simulink model "control_lab5_sim"  (R2022b)
settings: Solver=VariableStepAuto  StartTime=0.0  StopTime=10.0  RelTol=1e-3
values from neighbouring files (symbols this model uses):
  b = 3.5077e-6    (= 3.5077e-06)    [control_lab5.m]    (also in power_system_1.m = input('Enter any serial number:'))
  J = 3.2284e-6    (= 3.2284e-06)    [control_lab5.m]    (also in newton_rapshon.m = [H,L;M,N;]; newton_rapshon2.m = [H,L;M,N;])
  Ke = 0.0274    [control_lab5.m]
  Kt = 0.000274    [control_lab5.m]
  L = 2^n-1    (= 15)    [PCM__Code.m]    (also in control_lab5.m = 2.75e-06; newton_rapshon.m = zeros(n-1,n-1); newton_rapshon2.m = zeros(n-1,n-1-m))
  R = 19    [control_lab5.m]
settings Model: Creator=Asus  LastModifiedBy=Asus

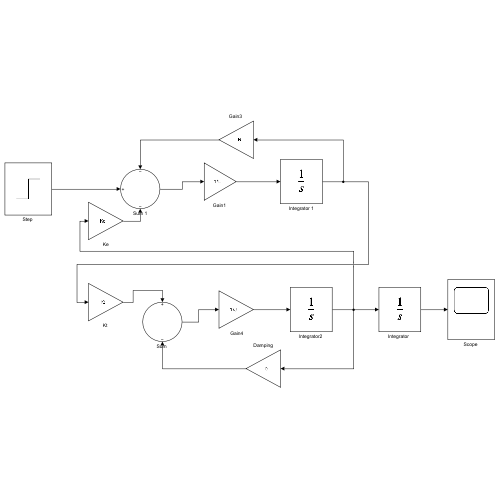
[thumbnail: Simulink's stored preview of the top-level diagram]
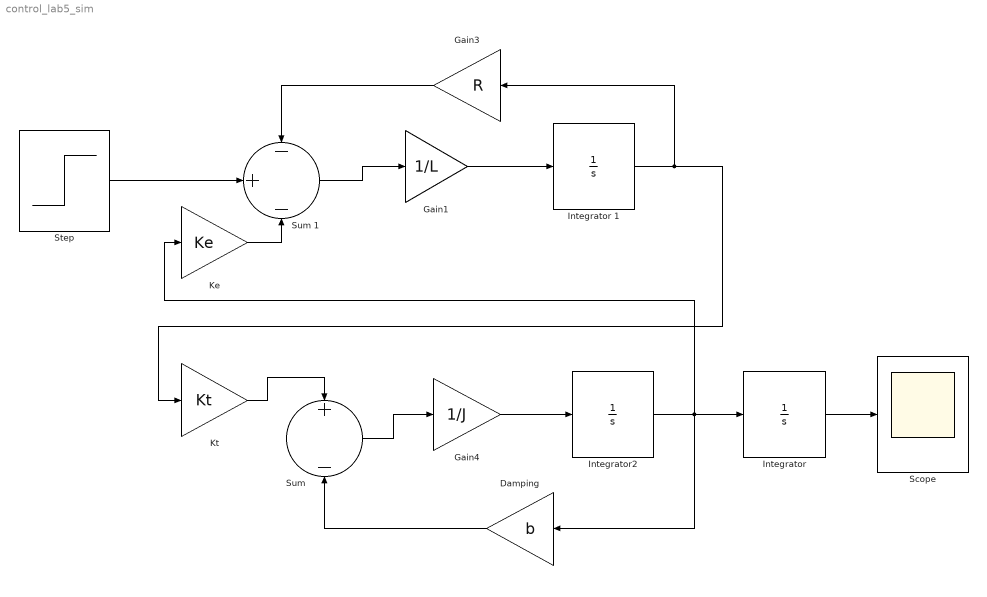
== system control_lab5_sim ==
  " Gain4" : Gain  Gain=1/J
  Damping : Gain  Gain=b
  "Gain1 " : Gain  Gain=1/L
  "Gain3 " : Gain  Gain=R
  "Integrator  " : Integrator
  Integrator 1 : Integrator
  "Integrator2 " : Integrator
  Ke : Gain  Gain=Ke
  "Kt " : Gain  Gain=Kt
  "Scope " : Scope
  "Step " : Step  SampleTime=0
  "Sum " : Sum  Inputs=+-
  Sum 1 : Sum  Inputs=-+-
  wires:
  "Step "/1 -> Sum 1/2
  "Gain3 "/1 -> Sum 1/1
  Ke/1 -> Sum 1/3
  Sum 1/1 -> "Gain1 "/1
  "Gain1 "/1 -> Integrator 1/1
  Integrator 1/1 -> "Kt "/1, "Gain3 "/1
  "Kt "/1 -> "Sum "/1
  Damping/1 -> "Sum "/2
  "Sum "/1 -> " Gain4"/1
  " Gain4"/1 -> "Integrator2 "/1
  "Integrator2 "/1 -> Ke/1, "Integrator  "/1, Damping/1
  "Integrator  "/1 -> "Scope "/1
